simulink model "ramadan_2022"  (R2021a)
settings: Solver=ode15s  StartTime=0.0  StopTime=10  MaxStep=1e-2  MinStep=1e-20  RelTol=1e-3
StartFcn:
  | tic
StopFcn:
  | toc
  | 
  | 
  | %if GimbalLockFlag
  |  % fprintf(2, 'Almost reached Gimbal Lock of IMU. Simulation stopped.\n')
  | %end
  | 
  | %fprintf('Elapsed time: %4.2f sec (%4.2f%% realtime)\n', a, tout(end)/a*100)
values from neighbouring files (symbols this model uses):
  Balance = pMod(26:29)    [AssignSimulinkParams.m]    (also in assign_parameters.m = param(26:29))
  BalanceTrunkLat = pMod(22:25)    [AssignSimulinkParams.m]    (also in assign_parameters.m = param(22:25))
  BasisStim = pMod(1:11)    [AssignSimulinkParams.m]    (also in assign_parameters.m = param(1:11))
  CompliantLeg = pMod(12:14)    [AssignSimulinkParams.m]    (also in assign_parameters.m = param(12:14))
  CompliantLegLat = pMod(15)    [AssignSimulinkParams.m]    (also in assign_parameters.m = param(15))
  lp1 = 0.45    [nms3D_prep.m]
  lp2 = 0.55    [nms3D_prep.m]
  N = size(x,1)    [cmaes_hg.m]
  PreventKneeOverextension = pMod(16:21)    [AssignSimulinkParams.m]    (also in assign_parameters.m = param(16:21))
  propulsion = pMod(35)    [AssignSimulinkParams.m]    (also in assign_parameters.m = param(35))
  s = x(1:N-1,:).^2 + x(2:N,:).^2    [cmaes_hg.m]
  Target02 = pMod(30)    [AssignSimulinkParams.m]    (also in assign_parameters.m = param(30))
  Target13 = pMod(31:33)    [AssignSimulinkParams.m]    (also in assign_parameters.m = param(31:33))
  theta0 = pMod(34)    [AssignSimulinkParams.m]    (also in assign_parameters.m = param(34))
  WramameiSL_1000 = readmatrix('WSL_1000_Norm_Sigmoid_MSE_cont.csv')    [nms3D_prep.m]
  ZramameiSL_1000 = readmatrix('ZSL_1000_Norm_Sigmoid_MSE_cont.csv')    [nms3D_prep.m]
undefined symbols (not defined in the file or in its folder): ICs, mParams, X, Y, Z
libraries: nesl_utility x110, sm_lib x88, simulink x79, eeGeneralControl x28, robotmaniplib x10, dspinverses x10, robotcorelib x5, dspmathops x3, pid_lib x2, vrlib x1
(part 2 of 9)

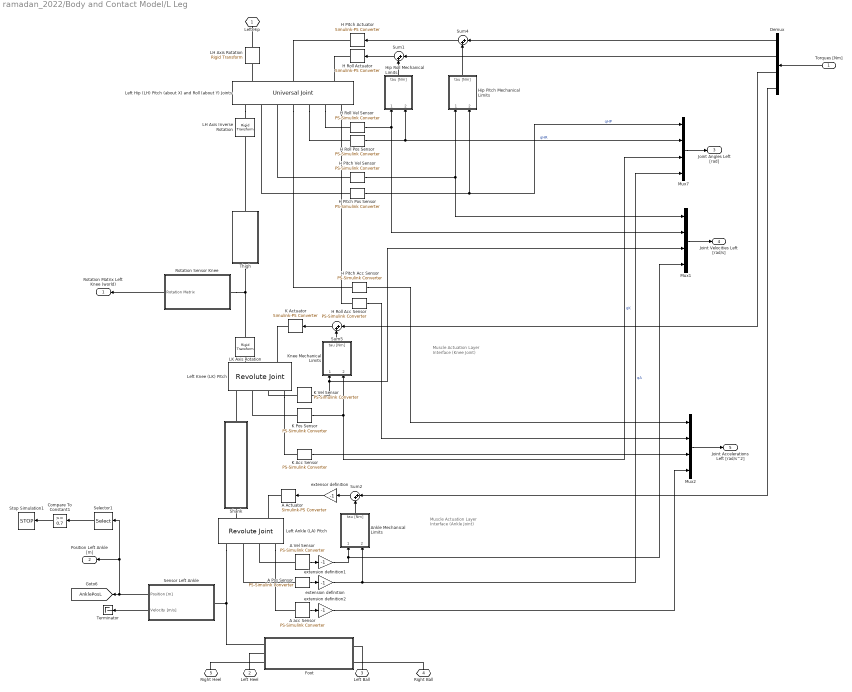
== system ramadan_2022/Body and Contact Model/L Leg ==
  note: Muscle Actuation
      | Layer Interface
      | (Ankle Joint)
  note: Muscle Actuation
      | Layer Interface
      | (Knee Joint)
  Torques [Nm] : Inport
  " K Actuator" : nesl_utility/Simulink-PS Converter  PhysicalDomain=network_engine_domain  SubClassName=ps_input  LeftPortType=input  RightPortType=output  PseudoPeriodic=off  Frequencies=[]  NoiseDistribution=none  NoiseParameters=[]  Unit=N*m  AffineConversion=off  FilteringAndDerivatives=zero  SimscapeFilterOrder=1  InputFilterTimeConstant=.001  UdotUserProvided=0
      settings: SourceProductBaseCode=PW,SS
  A Actuator : nesl_utility/Simulink-PS Converter  PhysicalDomain=network_engine_domain  SubClassName=ps_input  LeftPortType=input  RightPortType=output  PseudoPeriodic=off  Frequencies=[]  NoiseDistribution=none  NoiseParameters=[]  Unit=N*m  AffineConversion=off  FilteringAndDerivatives=zero  SimscapeFilterOrder=1  InputFilterTimeConstant=.001  UdotUserProvided=0
      settings: SourceProductBaseCode=PW,SS
  A Pos Sensor : nesl_utility/PS-Simulink Converter  PhysicalDomain=network_engine_domain  SubClassName=ps_output  LeftPortType=input  RightPortType=output  PseudoPeriodic=off  Frequencies=[]  Unit=rad  AffineConversion=off
      settings: SourceProductBaseCode=PW,SS
  A Vel Sensor : nesl_utility/PS-Simulink Converter  PhysicalDomain=network_engine_domain  SubClassName=ps_output  LeftPortType=input  RightPortType=output  PseudoPeriodic=off  Frequencies=[]  Unit=rad/s  AffineConversion=off
      settings: SourceProductBaseCode=PW,SS
  A acc Sensor : nesl_utility/PS-Simulink Converter  PhysicalDomain=network_engine_domain  SubClassName=ps_output  LeftPortType=input  RightPortType=output  PseudoPeriodic=off  Frequencies=[]  Unit=rad/(s^2)  AffineConversion=off
      settings: SourceProductBaseCode=PW,SS
  Ankle Mechanical Limits : Subsystem
  Compare To Constant1 : simulink/Logic and Bit Operations/Compare To Constant  relop=>=  const=0.7  OutDataTypeStr=boolean
  Demux : Demux
  Foot : Subsystem
  H Pitch Actuator : nesl_utility/Simulink-PS Converter  PhysicalDomain=network_engine_domain  SubClassName=ps_input  LeftPortType=input  RightPortType=output  PseudoPeriodic=off  Frequencies=[]  NoiseDistribution=none  NoiseParameters=[]  Unit=N*m  AffineConversion=off  FilteringAndDerivatives=zero  SimscapeFilterOrder=1  InputFilterTimeConstant=.001  UdotUserProvided=0
      settings: SourceProductBaseCode=PW,SS
  H Pitch Acc Sensor : nesl_utility/PS-Simulink Converter  PhysicalDomain=network_engine_domain  SubClassName=ps_output  LeftPortType=input  RightPortType=output  PseudoPeriodic=off  Frequencies=[]  Unit=rad/(s^2)  AffineConversion=off
      settings: SourceProductBaseCode=PW,SS
  H Pitch Pos Sensor : nesl_utility/PS-Simulink Converter  PhysicalDomain=network_engine_domain  SubClassName=ps_output  LeftPortType=input  RightPortType=output  PseudoPeriodic=off  Frequencies=[]  Unit=rad  AffineConversion=off
      settings: SourceProductBaseCode=PW,SS
  H Pitch Vel Sensor : nesl_utility/PS-Simulink Converter  PhysicalDomain=network_engine_domain  SubClassName=ps_output  LeftPortType=input  RightPortType=output  PseudoPeriodic=off  Frequencies=[]  Unit=rad/s  AffineConversion=off
      settings: SourceProductBaseCode=PW,SS
  H Roll Actuator : nesl_utility/Simulink-PS Converter  PhysicalDomain=network_engine_domain  SubClassName=ps_input  LeftPortType=input  RightPortType=output  PseudoPeriodic=off  Frequencies=[]  NoiseDistribution=none  NoiseParameters=[]  Unit=N*m  AffineConversion=off  FilteringAndDerivatives=zero  SimscapeFilterOrder=1  InputFilterTimeConstant=.001  UdotUserProvided=0
      settings: SourceProductBaseCode=PW,SS
  H Roll Acc Sensor : nesl_utility/PS-Simulink Converter  PhysicalDomain=network_engine_domain  SubClassName=ps_output  LeftPortType=input  RightPortType=output  PseudoPeriodic=off  Frequencies=[]  Unit=rad/(s^2)  AffineConversion=off
      settings: SourceProductBaseCode=PW,SS
  H Roll Pos Sensor : nesl_utility/PS-Simulink Converter  PhysicalDomain=network_engine_domain  SubClassName=ps_output  LeftPortType=input  RightPortType=output  PseudoPeriodic=off  Frequencies=[]  Unit=rad  AffineConversion=off
      settings: SourceProductBaseCode=PW,SS
  "H Roll Vel Sensor " : nesl_utility/PS-Simulink Converter  PhysicalDomain=network_engine_domain  SubClassName=ps_output  LeftPortType=input  RightPortType=output  PseudoPeriodic=off  Frequencies=[]  Unit=rad/s  AffineConversion=off
      settings: SourceProductBaseCode=PW,SS
  Hip Pitch Mechanical Limits : Subsystem
  Hip Roll Mechanical Limits : Subsystem
  K Acc Sensor : nesl_utility/PS-Simulink Converter  PhysicalDomain=network_engine_domain  SubClassName=ps_output  LeftPortType=input  RightPortType=output  PseudoPeriodic=off  Frequencies=[]  Unit=rad/(s^2)  AffineConversion=off
      settings: SourceProductBaseCode=PW,SS
  K Pos Sensor : nesl_utility/PS-Simulink Converter  PhysicalDomain=network_engine_domain  SubClassName=ps_output  LeftPortType=input  RightPortType=output  PseudoPeriodic=off  Frequencies=[]  Unit=rad  AffineConversion=off
      settings: SourceProductBaseCode=PW,SS
  K Vel Sensor : nesl_utility/PS-Simulink Converter  PhysicalDomain=network_engine_domain  SubClassName=ps_output  LeftPortType=input  RightPortType=output  PseudoPeriodic=off  Frequencies=[]  Unit=rad/s  AffineConversion=off
      settings: SourceProductBaseCode=PW,SS
  Knee Mechanical Limits : Subsystem
  LH Axis Inverse Rotation : sm_lib/Frames and Transforms/Rigid Transform  TranslationMethod=None  TranslationStandardOffset=-0.2  TranslationLengthUnit=m  TranslationStandardAxis=+Y  TranslationCartesianOffset=0  TranslationROffset=0  TranslationROffsetUnits=m  TranslationZOffset=0  TranslationZOffsetUnits=m  TranslationThetaOffset=0  TranslationThetaOffsetUnits=deg  RotationMethod=RotationSequence  RotationAngleUnits=deg  RotationStandardAxis=+X  RotationAngle=-90  RotationArbitraryAxis=[0 0 1]  FollAlignAxisA=+X  BaseAlignAxisA=+Y  FollAlignAxisB=+Y  BaseAlignAxisB=+Z  RotationSequenceAxes=BaseAxes  RotationSequence=YXY  RotationSequenceAngles=[-90 -90 0]  RotationSequenceAnglesUnits=deg  RotationMatrix=[1 0 0; 0 1 0; 0 0 1]
  LH Axis Rotation : sm_lib/Frames and Transforms/Rigid Transform  TranslationMethod=None  TranslationStandardOffset=-0.2  TranslationLengthUnit=m  TranslationStandardAxis=+Y  TranslationCartesianOffset=0  TranslationROffset=0  TranslationROffsetUnits=m  TranslationZOffset=0  TranslationZOffsetUnits=m  TranslationThetaOffset=0  TranslationThetaOffsetUnits=deg  RotationMethod=RotationSequence  RotationAngleUnits=deg  RotationStandardAxis=+X  RotationAngle=90  RotationArbitraryAxis=[0 0 1]  FollAlignAxisA=+X  BaseAlignAxisA=+Y  FollAlignAxisB=+Y  BaseAlignAxisB=+Z  RotationSequenceAxes=FollowerAxes  RotationSequence=XZX  RotationSequenceAngles=[-90 90 0]  RotationSequenceAnglesUnits=deg  RotationMatrix=[1 0 0; 0 1 0; 0 0 1]
  LK Axis Rotation : sm_lib/Frames and Transforms/Rigid Transform  TranslationMethod=None  TranslationStandardOffset=-0.5  TranslationLengthUnit=m  TranslationStandardAxis=+Y  TranslationCartesianOffset=0  TranslationROffset=0  TranslationROffsetUnits=m  TranslationZOffset=0  TranslationZOffsetUnits=m  TranslationThetaOffset=0  TranslationThetaOffsetUnits=deg  RotationMethod=RotationSequence  RotationAngleUnits=deg  RotationStandardAxis=+X  RotationAngle=-90  RotationArbitraryAxis=[0 0 1]  FollAlignAxisA=+X  BaseAlignAxisA=+Y  FollAlignAxisB=+Y  BaseAlignAxisB=+Z  RotationSequenceAxes=BaseAxes  RotationSequence=ZXZ  RotationSequenceAngles=[180 0 0]  RotationSequenceAnglesUnits=deg  RotationMatrix=[1 0 0; 0 1 0; 0 0 1]
  Left Ankle (LA) Pitch : sm_lib/Joints/Revolute Joint  JointMode=Normal  SenseConstraintForce=off  SenseConstraintForceX=off  SenseConstraintForceY=off  SenseConstraintForceZ=off  SenseConstraintTorque=off  SenseConstraintTorqueX=off  SenseConstraintTorqueY=off  SenseConstraintTorqueZ=off  SenseTotalForce=off  SenseTotalForceX=off  SenseTotalForceY=off  SenseTotalForceZ=off  SenseTotalTorque=off  SenseTotalTorqueX=off  SenseTotalTorqueY=off  SenseTotalTorqueZ=off  CompositeWrenchDir=FollowerOnBase  CompositeWrenchFrame=FollowerFrame  EquilibriumPosition=0  EquilibriumPositionUnits=deg  SpringStiffness=0  SpringStiffnessUnits=N*m/deg  DampingCoefficient=0  DampingCoefficientUnits=N*m/(deg/s)  TorqueActuationMode=InputTorque  MotionActuationMode=ComputedMotion  SensePosition=on  SenseVelocity=on  SenseAcceleration=on  SenseTorqueForce=off  SenseLowerLimitTorqueForce=off  SenseUpperLimitTorqueForce=off  LowerLimitSpecify=off  LowerLimitBound=-90  LowerLimitBoundUnits=deg  LowerLimitStiffness=1e4  LowerLimitStiffnessUnits=N*m/deg  LowerLimitDamping=10  LowerLimitDampingUnits=N*m/(deg/s)  LowerLimitTransitionRegionWidth=0.1  LowerLimitTransitionRegionWidthUnits=deg  UpperLimitSpecify=off  UpperLimitBound=90  UpperLimitBoundUnits=deg  UpperLimitStiffness=1e4  UpperLimitStiffnessUnits=N*m/deg  UpperLimitDamping=10  UpperLimitDampingUnits=N*m/(deg/s)  UpperLimitTransitionRegionWidth=0.1  UpperLimitTransitionRegionWidthUnits=deg  PositionTargetSpecify=on  PositionTargetPriority=High  PositionTargetValue=-ICs.lLeg.ankle.qP0  PositionTargetValueUnits=rad  VelocityTargetSpecify=on  VelocityTargetPriority=High  VelocityTargetValue=0  VelocityTargetValueUnits=rad/s
  Left Hip (LH) Pitch (about X) and Roll (about Y) Joints : sm_lib/Joints/Universal Joint  JointMode=Normal  SenseConstraintForce=off  SenseConstraintForceX=off  SenseConstraintForceY=off  SenseConstraintForceZ=off  SenseConstraintTorque=off  SenseConstraintTorqueX=off  SenseConstraintTorqueY=off  SenseConstraintTorqueZ=off  SenseTotalForce=off  SenseTotalForceX=off  SenseTotalForceY=off  SenseTotalForceZ=off  SenseTotalTorque=off  SenseTotalTorqueX=off  SenseTotalTorqueY=off  SenseTotalTorqueZ=off  CompositeWrenchDir=FollowerOnBase  CompositeWrenchFrame=FollowerFrame  RxEquilibriumPosition=0  RxEquilibriumPositionUnits=deg  RxSpringStiffness=0  RxSpringStiffnessUnits=N*m/deg  RxDampingCoefficient=0  RxDampingCoefficientUnits=N*m/(deg/s)  RxTorqueActuationMode=InputTorque  RxMotionActuationMode=ComputedMotion  RxSensePosition=on  RxSenseVelocity=on  RxSenseAcceleration=on  RxSenseTorqueForce=off  RxSenseLowerLimitTorqueForce=off  RxSenseUpperLimitTorqueForce=off  RxLowerLimitSpecify=off  RxLowerLimitBound=-90  RxLowerLimitBoundUnits=deg  RxLowerLimitStiffness=1e4  RxLowerLimitStiffnessUnits=N*m/deg  RxLowerLimitDamping=10  RxLowerLimitDampingUnits=N*m/(deg/s)  RxLowerLimitTransitionRegionWidth=0.1  RxLowerLimitTransitionRegionWidthUnits=deg  RxUpperLimitSpecify=off  RxUpperLimitBound=90  RxUpperLimitBoundUnits=deg  RxUpperLimitStiffness=1e4  RxUpperLimitStiffnessUnits=N*m/deg  RxUpperLimitDamping=10  RxUpperLimitDampingUnits=N*m/(deg/s)  RxUpperLimitTransitionRegionWidth=0.1  RxUpperLimitTransitionRegionWidthUnits=deg  RxPositionTargetSpecify=on  RxPositionTargetPriority=High  RxPositionTargetValue=ICs.lLeg.hip.qP0  RxPositionTargetValueUnits=rad  RxVelocityTargetSpecify=on  RxVelocityTargetPriority=High  RxVelocityTargetValue=0  RxVelocityTargetValueUnits=rad/s  RyEquilibriumPosition=0  RyEquilibriumPositionUnits=deg  RySpringStiffness=0  RySpringStiffnessUnits=N*m/deg  RyDampingCoefficient=0  RyDampingCoefficientUnits=N*m/(deg/s)  RyTorqueActuationMode=InputTorque  RyMotionActuationMode=ComputedMotion  RySensePosition=on  RySenseVelocity=on  RySenseAcceleration=on  RySenseTorqueForce=off  RySenseLowerLimitTorqueForce=off  RySenseUpperLimitTorqueForce=off  RyLowerLimitSpecify=off  RyLowerLimitBound=-90  RyLowerLimitBoundUnits=deg  RyLowerLimitStiffness=1e4  RyLowerLimitStiffnessUnits=N*m/deg  RyLowerLimitDamping=10  RyLowerLimitDampingUnits=N*m/(deg/s)  RyLowerLimitTransitionRegionWidth=0.1  RyLowerLimitTransitionRegionWidthUnits=deg  RyUpperLimitSpecify=off  RyUpperLimitBound=90  RyUpperLimitBoundUnits=deg  RyUpperLimitStiffness=1e4  RyUpperLimitStiffnessUnits=N*m/deg  RyUpperLimitDamping=10  RyUpperLimitDampingUnits=N*m/(deg/s)  RyUpperLimitTransitionRegionWidth=0.1  RyUpperLimitTransitionRegionWidthUnits=deg  RyPositionTargetSpecify=on  RyPositionTargetPriority=High  RyPositionTargetValue=ICs.lLeg.hip.qR0  RyPositionTargetValueUnits=rad  RyVelocityTargetSpecify=on  RyVelocityTargetPriority=High  RyVelocityTargetValue=0  RyVelocityTargetValueUnits=rad/s
  Left Knee (LK) Pitch : sm_lib/Joints/Revolute Joint  JointMode=Normal  SenseConstraintForce=off  SenseConstraintForceX=off  SenseConstraintForceY=off  SenseConstraintForceZ=off  SenseConstraintTorque=off  SenseConstraintTorqueX=off  SenseConstraintTorqueY=off  SenseConstraintTorqueZ=off  SenseTotalForce=off  SenseTotalForceX=off  SenseTotalForceY=off  SenseTotalForceZ=off  SenseTotalTorque=off  SenseTotalTorqueX=off  SenseTotalTorqueY=off  SenseTotalTorqueZ=off  CompositeWrenchDir=FollowerOnBase  CompositeWrenchFrame=FollowerFrame  EquilibriumPosition=0  EquilibriumPositionUnits=deg  SpringStiffness=0  SpringStiffnessUnits=N*m/deg  DampingCoefficient=0  DampingCoefficientUnits=N*m/(deg/s)  TorqueActuationMode=InputTorque  MotionActuationMode=ComputedMotion  SensePosition=on  SenseVelocity=on  SenseAcceleration=on  SenseTorqueForce=off  SenseLowerLimitTorqueForce=off  SenseUpperLimitTorqueForce=off  LowerLimitSpecify=off  LowerLimitBound=-90  LowerLimitBoundUnits=deg  LowerLimitStiffness=1e4  LowerLimitStiffnessUnits=N*m/deg  LowerLimitDamping=10  LowerLimitDampingUnits=N*m/(deg/s)  LowerLimitTransitionRegionWidth=0.1  LowerLimitTransitionRegionWidthUnits=deg  UpperLimitSpecify=off  UpperLimitBound=90  UpperLimitBoundUnits=deg  UpperLimitStiffness=1e4  UpperLimitStiffnessUnits=N*m/deg  UpperLimitDamping=10  UpperLimitDampingUnits=N*m/(deg/s)  UpperLimitTransitionRegionWidth=0.1  UpperLimitTransitionRegionWidthUnits=deg  PositionTargetSpecify=on  PositionTargetPriority=High  PositionTargetValue=ICs.lLeg.knee.qP0  PositionTargetValueUnits=rad  VelocityTargetSpecify=on  VelocityTargetPriority=High  VelocityTargetValue=0  VelocityTargetValueUnits=rad/s
  Mux1 : Mux
  Mux2 : Mux
  Mux7 : Mux
  Rotation Sensor Knee : Subsystem
  Selector1 : Selector  InputPortWidth=3  IndexOptions=Index vector (dialog)  Indices=[2]  OutputSizes=1
  Sensor Left Ankle : Subsystem
  Shank : Subsystem
  Stop Simulation1 : Stop
  Sum{1..2,4..5} (4 alike) : Sum  Inputs=|++
  Terminator : Terminator
  Thigh : Subsystem
  extension definition : Gain  Gain=-1
  extension definition1 : Gain  Gain=-1
  extension definition2 : Gain  Gain=-1
  extensor definition : Gain  Gain=-1
  Left Hip : PMIOPort  Side=Left
  Left Heel : PMIOPort  Port=2  Side=Right
  Left Ball : PMIOPort  Port=3  Side=Right
  Right Ball : PMIOPort  Port=4  Side=Right
  Right Heel : PMIOPort  Port=5  Side=Right
  Rotation Matrix Left Knee (world) : Outport
  " Position Left Ankle [m]" : Outport  Port=2
  Joint Angles Left [rad] : Outport  Port=3
  "Joint Velocities Left [rad/s] " : Outport  Port=4
  Joint Accelerations Left [rad/s^2] : Outport  Port=5
  tag scope: AnklePosL=global
  wires:
  extension definition1/1 -> Mux1/4, Ankle Mechanical Limits/1(dq [rad/s])
  A Pos Sensor/1 -> extension definition/1
  Ankle Mechanical Limits/1(tau [Nm]) -> Sum2/2
  A Vel Sensor/1 -> extension definition1/1
  Sum2/1 -> extensor definition/1
  "H Roll Vel Sensor "/1 -> Mux1/2, Hip Roll Mechanical Limits/1(dq [rad/s])
  K Vel Sensor/1 -> Mux1/3, Knee Mechanical Limits/1(dq [rad/s])
  Knee Mechanical Limits/1(tau [Nm]) -> Sum5/2
  Hip Roll Mechanical Limits/1(tau [Nm]) -> Sum1/2
  H Pitch Vel Sensor/1 -> Mux1/1, Hip Pitch Mechanical Limits/1(dq [rad/s])
  Hip Pitch Mechanical Limits/1(tau [Nm]) -> Sum4/2
  Sum4/1 -> H Pitch Actuator/1
  Sum1/1 -> H Roll Actuator/1
  Sum5/1 -> " K Actuator"/1
  extensor definition/1 -> A Actuator/1
  Mux1/1 -> "Joint Velocities Left [rad/s] "/1
  Mux2/1 -> Joint Accelerations Left [rad/s^2]/1
  H Pitch Acc Sensor/1 -> Mux2/1
  H Roll Acc Sensor/1 -> Mux2/2
  K Acc Sensor/1 -> Mux2/3
  A acc Sensor/1 -> extension definition2/1
  extension definition2/1 -> Mux2/4
  Demux/1 -> Sum4/1
  Demux/2 -> Sum1/1
  Demux/3 -> Sum5/1
  Demux/4 -> Sum2/1
  Sensor Left Ankle/1(Position [m]) -> " Position Left Ankle [m]"/1, Selector1/1, [AnklePosL]
  Rotation Sensor Knee/1(Rotation Matrix) -> Rotation Matrix Left Knee (world)/1
  Sensor Left Ankle/2(Velocity [m/s]) -> Terminator/1
  Torques [Nm]/1 -> Demux/1
  K Pos Sensor/1 -> Mux7/3, Knee Mechanical Limits/2(q [rad])  "qK"
  H Pitch Pos Sensor/1 -> Hip Pitch Mechanical Limits/2(q [rad]), Mux7/1  "qHP"
  H Roll Pos Sensor/1 -> Mux7/2, Hip Roll Mechanical Limits/2(q [rad])  "qHR"
  extension definition/1 -> Mux7/4, Ankle Mechanical Limits/2(q [rad])  "qA"
  Mux7/1 -> Joint Angles Left [rad]/1
  Selector1/1 -> Compare To Constant1/1
  Compare To Constant1/1 -> Stop Simulation1/1
  connections:
  Left Ankle (LA) Pitch/RConn1 -- Sensor Left Ankle/LConn1 -- Foot/LConn1
  A Pos Sensor/LConn1 -- Left Ankle (LA) Pitch/RConn2
  A Vel Sensor/LConn1 -- Left Ankle (LA) Pitch/RConn3
  Left Ankle (LA) Pitch/LConn1 -- Shank/RConn1
  Left Hip (LH) Pitch (about X) and Roll (about Y) Joints/RConn1 -- LH Axis Inverse Rotation/LConn1
  Thigh/RConn1 -- Rotation Sensor Knee/LConn1 -- LK Axis Rotation/LConn1
  Shank/LConn1 -- Left Knee (LK) Pitch/RConn1
  Left Hip (LH) Pitch (about X) and Roll (about Y) Joints/LConn1 -- LH Axis Rotation/RConn1
  H Pitch Vel Sensor/LConn1 -- Left Hip (LH) Pitch (about X) and Roll (about Y) Joints/RConn3
  H Pitch Pos Sensor/LConn1 -- Left Hip (LH) Pitch (about X) and Roll (about Y) Joints/RConn2
  K Pos Sensor/LConn1 -- Left Knee (LK) Pitch/RConn2
  K Vel Sensor/LConn1 -- Left Knee (LK) Pitch/RConn3
  LH Axis Rotation/LConn1 -- Left Hip/RConn1
  Left Hip (LH) Pitch (about X) and Roll (about Y) Joints/RConn6 -- "H Roll Vel Sensor "/LConn1
  Left Hip (LH) Pitch (about X) and Roll (about Y) Joints/RConn5 -- H Roll Pos Sensor/LConn1
  Left Hip (LH) Pitch (about X) and Roll (about Y) Joints/RConn4 -- H Pitch Acc Sensor/LConn1
  Left Hip (LH) Pitch (about X) and Roll (about Y) Joints/RConn7 -- H Roll Acc Sensor/LConn1
  Left Knee (LK) Pitch/RConn4 -- K Acc Sensor/LConn1
  Left Ankle (LA) Pitch/RConn4 -- A acc Sensor/LConn1
  LK Axis Rotation/RConn1 -- Left Knee (LK) Pitch/LConn1
  Right Heel/RConn1 -- Foot/LConn3
  Foot/LConn2 -- Left Heel/RConn1
  Left Ball/RConn1 -- Foot/RConn1
  Right Ball/RConn1 -- Foot/RConn2
  Thigh/LConn1 -- LH Axis Inverse Rotation/RConn1
  " K Actuator"/RConn1 -- Left Knee (LK) Pitch/LConn2
  A Actuator/RConn1 -- Left Ankle (LA) Pitch/LConn2
  H Pitch Actuator/RConn1 -- Left Hip (LH) Pitch (about X) and Roll (about Y) Joints/LConn2
  H Roll Actuator/RConn1 -- Left Hip (LH) Pitch (about X) and Roll (about Y) Joints/LConn3

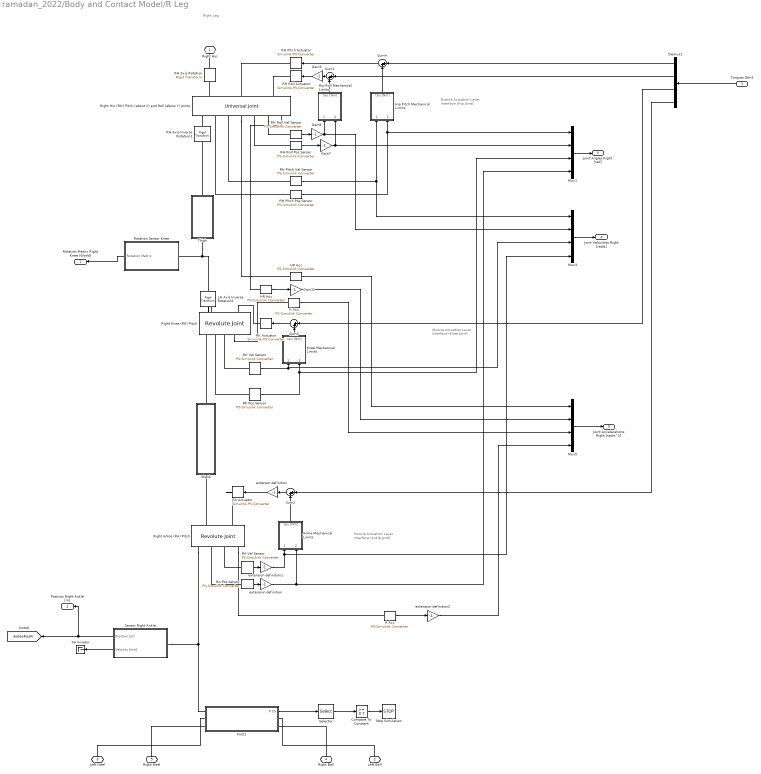
== system ramadan_2022/Body and Contact Model/R Leg ==
  note: Muscle Actuation
      | Layer Interface
      | (Hip Joint)
  note: Muscle Actuation
      | Layer Interface
      | (Knee Joint)
  note: Muscle Actuation
      | Layer Interface
      | (Ankle Joint)
  note: Right Leg
  Torques [Nm] : Inport
  A Acc : nesl_utility/PS-Simulink Converter  PhysicalDomain=network_engine_domain  SubClassName=ps_output  LeftPortType=input  RightPortType=output  PseudoPeriodic=off  Frequencies=[]  Unit=rad/(s^2)  AffineConversion=off
      settings: SourceProductBaseCode=PW,SS
  Ankle Mechanical Limits : Subsystem
  Compare To Constant : simulink/Logic and Bit Operations/Compare To Constant  relop=>=  const=0.7  OutDataTypeStr=boolean
  Demux1 : Demux
  Foot1 : Subsystem
  Gain{3,7..8,11} (4 alike) : Gain  Gain=-1
  HP Acc : nesl_utility/PS-Simulink Converter  PhysicalDomain=network_engine_domain  SubClassName=ps_output  LeftPortType=input  RightPortType=output  PseudoPeriodic=off  Frequencies=[]  Unit=rad/(s^2)  AffineConversion=off
      settings: SourceProductBaseCode=PW,SS
  HR Acc : nesl_utility/PS-Simulink Converter  PhysicalDomain=network_engine_domain  SubClassName=ps_output  LeftPortType=input  RightPortType=output  PseudoPeriodic=off  Frequencies=[]  Unit=rad/(s^2)  AffineConversion=off
      settings: SourceProductBaseCode=PW,SS
  Hip Pitch Mechanical Limits : Subsystem
  Hip Roll Mechanical Limits : Subsystem
  K Acc : nesl_utility/PS-Simulink Converter  PhysicalDomain=network_engine_domain  SubClassName=ps_output  LeftPortType=input  RightPortType=output  PseudoPeriodic=off  Frequencies=[]  Unit=rad/(s^2)  AffineConversion=off
      settings: SourceProductBaseCode=PW,SS
  Knee Mechanical Limits : Subsystem
  LH Axis Inverse Rotation1 : sm_lib/Frames and Transforms/Rigid Transform  TranslationMethod=None  TranslationStandardOffset=-0.5  TranslationLengthUnit=m  TranslationStandardAxis=+Y  TranslationCartesianOffset=0  TranslationROffset=0  TranslationROffsetUnits=m  TranslationZOffset=0  TranslationZOffsetUnits=m  TranslationThetaOffset=0  TranslationThetaOffsetUnits=deg  RotationMethod=RotationSequence  RotationAngleUnits=deg  RotationStandardAxis=+X  RotationAngle=-90  RotationArbitraryAxis=[0 0 1]  FollAlignAxisA=+X  BaseAlignAxisA=+Y  FollAlignAxisB=+Y  BaseAlignAxisB=+Z  RotationSequenceAxes=BaseAxes  RotationSequence=ZXZ  RotationSequenceAngles=[180 0 0]  RotationSequenceAnglesUnits=deg  RotationMatrix=[1 0 0; 0 1 0; 0 0 1]
  Mux1 : Mux
  Mux3 : Mux
  Mux5 : Mux
  RA Actuator : nesl_utility/Simulink-PS Converter  PhysicalDomain=network_engine_domain  SubClassName=ps_input  LeftPortType=input  RightPortType=output  PseudoPeriodic=off  Frequencies=[]  NoiseDistribution=none  NoiseParameters=[]  Unit=N*m  AffineConversion=off  FilteringAndDerivatives=zero  SimscapeFilterOrder=1  InputFilterTimeConstant=.001  UdotUserProvided=0
      settings: SourceProductBaseCode=PW,SS
  RA Pos Sensor : nesl_utility/PS-Simulink Converter  PhysicalDomain=network_engine_domain  SubClassName=ps_output  LeftPortType=input  RightPortType=output  PseudoPeriodic=off  Frequencies=[]  Unit=rad  AffineConversion=off
      settings: SourceProductBaseCode=PW,SS
  RA Vel Sensor : nesl_utility/PS-Simulink Converter  PhysicalDomain=network_engine_domain  SubClassName=ps_output  LeftPortType=input  RightPortType=output  PseudoPeriodic=off  Frequencies=[]  Unit=rad/s  AffineConversion=off
      settings: SourceProductBaseCode=PW,SS
  RH Pitch Pos Sensor : nesl_utility/PS-Simulink Converter  PhysicalDomain=network_engine_domain  SubClassName=ps_output  LeftPortType=input  RightPortType=output  PseudoPeriodic=off  Frequencies=[]  Unit=rad  AffineConversion=off
      settings: SourceProductBaseCode=PW,SS
  RH Pitch Vel Sensor : nesl_utility/PS-Simulink Converter  PhysicalDomain=network_engine_domain  SubClassName=ps_output  LeftPortType=input  RightPortType=output  PseudoPeriodic=off  Frequencies=[]  Unit=rad/s  AffineConversion=off
      settings: SourceProductBaseCode=PW,SS
  RH Roll Pos Sensor : nesl_utility/PS-Simulink Converter  PhysicalDomain=network_engine_domain  SubClassName=ps_output  LeftPortType=input  RightPortType=output  PseudoPeriodic=off  Frequencies=[]  Unit=rad  AffineConversion=off
      settings: SourceProductBaseCode=PW,SS
  "RH Roll Vel Sensor " : nesl_utility/PS-Simulink Converter  PhysicalDomain=network_engine_domain  SubClassName=ps_output  LeftPortType=input  RightPortType=output  PseudoPeriodic=off  Frequencies=[]  Unit=rad/s  AffineConversion=off
      settings: SourceProductBaseCode=PW,SS
  RH Axis Inverse Rotation1 : sm_lib/Frames and Transforms/Rigid Transform  TranslationMethod=None  TranslationStandardOffset=-0.5  TranslationLengthUnit=m  TranslationStandardAxis=+Y  TranslationCartesianOffset=[0 0.2 0]  TranslationROffset=0  TranslationROffsetUnits=m  TranslationZOffset=0  TranslationZOffsetUnits=m  TranslationThetaOffset=0  TranslationThetaOffsetUnits=deg  RotationMethod=RotationSequence  RotationAngleUnits=deg  RotationStandardAxis=+X  RotationAngle=-90  RotationArbitraryAxis=[0 0 1]  FollAlignAxisA=+X  BaseAlignAxisA=+Y  FollAlignAxisB=+Y  BaseAlignAxisB=+Z  RotationSequenceAxes=BaseAxes  RotationSequence=YXY  RotationSequenceAngles=[ -90 -90 0]  RotationSequenceAnglesUnits=deg  RotationMatrix=[1 0 0; 0 1 0; 0 0 1]
  RH Axis Rotation : sm_lib/Frames and Transforms/Rigid Transform  TranslationMethod=None  TranslationStandardOffset=-0  TranslationLengthUnit=m  TranslationStandardAxis=+Y  TranslationCartesianOffset=0  TranslationROffset=0  TranslationROffsetUnits=m  TranslationZOffset=0  TranslationZOffsetUnits=m  TranslationThetaOffset=0  TranslationThetaOffsetUnits=deg  RotationMethod=RotationSequence  RotationAngleUnits=deg  RotationStandardAxis=+X  RotationAngle=90  RotationArbitraryAxis=[0 0 1]  FollAlignAxisA=+X  BaseAlignAxisA=+Y  FollAlignAxisB=+Y  BaseAlignAxisB=+Z  RotationSequenceAxes=FollowerAxes  RotationSequence=XZX  RotationSequenceAngles=[-90 90 0]  RotationSequenceAnglesUnits=deg  RotationMatrix=[1 0 0; 0 1 0; 0 0 1]
  RH Pitch Actuator : nesl_utility/Simulink-PS Converter  PhysicalDomain=network_engine_domain  SubClassName=ps_input  LeftPortType=input  RightPortType=output  PseudoPeriodic=off  Frequencies=[]  NoiseDistribution=none  NoiseParameters=[]  Unit=N*m  AffineConversion=off  FilteringAndDerivatives=zero  SimscapeFilterOrder=1  InputFilterTimeConstant=.001  UdotUserProvided=0
      settings: SourceProductBaseCode=PW,SS
  RH Roll Actuator : nesl_utility/Simulink-PS Converter  PhysicalDomain=network_engine_domain  SubClassName=ps_input  LeftPortType=input  RightPortType=output  PseudoPeriodic=off  Frequencies=[]  NoiseDistribution=none  NoiseParameters=[]  Unit=N*m  AffineConversion=off  FilteringAndDerivatives=zero  SimscapeFilterOrder=1  InputFilterTimeConstant=.001  UdotUserProvided=0
      settings: SourceProductBaseCode=PW,SS
  RK Actuator : nesl_utility/Simulink-PS Converter  PhysicalDomain=network_engine_domain  SubClassName=ps_input  LeftPortType=input  RightPortType=output  PseudoPeriodic=off  Frequencies=[]  NoiseDistribution=none  NoiseParameters=[]  Unit=N*m  AffineConversion=off  FilteringAndDerivatives=zero  SimscapeFilterOrder=1  InputFilterTimeConstant=.001  UdotUserProvided=0
      settings: SourceProductBaseCode=PW,SS
  RK Pos Sensor : nesl_utility/PS-Simulink Converter  PhysicalDomain=network_engine_domain  SubClassName=ps_output  LeftPortType=input  RightPortType=output  PseudoPeriodic=off  Frequencies=[]  Unit=rad  AffineConversion=off
      settings: SourceProductBaseCode=PW,SS
  RK Vel Sensor : nesl_utility/PS-Simulink Converter  PhysicalDomain=network_engine_domain  SubClassName=ps_output  LeftPortType=input  RightPortType=output  PseudoPeriodic=off  Frequencies=[]  Unit=rad/s  AffineConversion=off
      settings: SourceProductBaseCode=PW,SS
  Right Ankle (RA) Pitch : sm_lib/Joints/Revolute Joint  JointMode=Normal  SenseConstraintForce=off  SenseConstraintForceX=off  SenseConstraintForceY=off  SenseConstraintForceZ=off  SenseConstraintTorque=off  SenseConstraintTorqueX=off  SenseConstraintTorqueY=off  SenseConstraintTorqueZ=off  SenseTotalForce=off  SenseTotalForceX=off  SenseTotalForceY=off  SenseTotalForceZ=off  SenseTotalTorque=off  SenseTotalTorqueX=off  SenseTotalTorqueY=off  SenseTotalTorqueZ=off  CompositeWrenchDir=FollowerOnBase  CompositeWrenchFrame=FollowerFrame  EquilibriumPosition=0  EquilibriumPositionUnits=deg  SpringStiffness=0  SpringStiffnessUnits=N*m/deg  DampingCoefficient=0  DampingCoefficientUnits=N*m/(deg/s)  TorqueActuationMode=InputTorque  MotionActuationMode=ComputedMotion  SensePosition=on  SenseVelocity=on  SenseAcceleration=on  SenseTorqueForce=off  SenseLowerLimitTorqueForce=off  SenseUpperLimitTorqueForce=off  LowerLimitSpecify=off  LowerLimitBound=-90  LowerLimitBoundUnits=deg  LowerLimitStiffness=1e4  LowerLimitStiffnessUnits=N*m/deg  LowerLimitDamping=10  LowerLimitDampingUnits=N*m/(deg/s)  LowerLimitTransitionRegionWidth=0.1  LowerLimitTransitionRegionWidthUnits=deg  UpperLimitSpecify=off  UpperLimitBound=90  UpperLimitBoundUnits=deg  UpperLimitStiffness=1e4  UpperLimitStiffnessUnits=N*m/deg  UpperLimitDamping=10  UpperLimitDampingUnits=N*m/(deg/s)  UpperLimitTransitionRegionWidth=0.1  UpperLimitTransitionRegionWidthUnits=deg  PositionTargetSpecify=on  PositionTargetPriority=High  PositionTargetValue=-ICs.rLeg.ankle.qP0  PositionTargetValueUnits=rad  VelocityTargetSpecify=on  VelocityTargetPriority=High  VelocityTargetValue=0  VelocityTargetValueUnits=rad/s
  Right Hip (RH) Pitch (about X) and Roll (about Y) Joints : sm_lib/Joints/Universal Joint  JointMode=Normal  SenseConstraintForce=off  SenseConstraintForceX=off  SenseConstraintForceY=off  SenseConstraintForceZ=off  SenseConstraintTorque=off  SenseConstraintTorqueX=off  SenseConstraintTorqueY=off  SenseConstraintTorqueZ=off  SenseTotalForce=off  SenseTotalForceX=off  SenseTotalForceY=off  SenseTotalForceZ=off  SenseTotalTorque=off  SenseTotalTorqueX=off  SenseTotalTorqueY=off  SenseTotalTorqueZ=off  CompositeWrenchDir=FollowerOnBase  CompositeWrenchFrame=FollowerFrame  RxEquilibriumPosition=0  RxEquilibriumPositionUnits=deg  RxSpringStiffness=0  RxSpringStiffnessUnits=N*m/deg  RxDampingCoefficient=0  RxDampingCoefficientUnits=N*m/(deg/s)  RxTorqueActuationMode=InputTorque  RxMotionActuationMode=ComputedMotion  RxSensePosition=on  RxSenseVelocity=on  RxSenseAcceleration=on  RxSenseTorqueForce=off  RxSenseLowerLimitTorqueForce=off  RxSenseUpperLimitTorqueForce=off  RxLowerLimitSpecify=off  RxLowerLimitBound=-90  RxLowerLimitBoundUnits=deg  RxLowerLimitStiffness=1e4  RxLowerLimitStiffnessUnits=N*m/deg  RxLowerLimitDamping=10  RxLowerLimitDampingUnits=N*m/(deg/s)  RxLowerLimitTransitionRegionWidth=0.1  RxLowerLimitTransitionRegionWidthUnits=deg  RxUpperLimitSpecify=off  RxUpperLimitBound=90  RxUpperLimitBoundUnits=deg  RxUpperLimitStiffness=1e4  RxUpperLimitStiffnessUnits=N*m/deg  RxUpperLimitDamping=10  RxUpperLimitDampingUnits=N*m/(deg/s)  RxUpperLimitTransitionRegionWidth=0.1  RxUpperLimitTransitionRegionWidthUnits=deg  RxPositionTargetSpecify=on  RxPositionTargetPriority=High  RxPositionTargetValue=ICs.rLeg.hip.qP0  RxPositionTargetValueUnits=rad  RxVelocityTargetSpecify=on  RxVelocityTargetPriority=High  RxVelocityTargetValue=0  RxVelocityTargetValueUnits=rad/s  RyEquilibriumPosition=0  RyEquilibriumPositionUnits=deg  RySpringStiffness=0  RySpringStiffnessUnits=N*m/deg  RyDampingCoefficient=0  RyDampingCoefficientUnits=N*m/(deg/s)  RyTorqueActuationMode=InputTorque  RyMotionActuationMode=ComputedMotion  RySensePosition=on  RySenseVelocity=on  RySenseAcceleration=on  RySenseTorqueForce=off  RySenseLowerLimitTorqueForce=off  RySenseUpperLimitTorqueForce=off  RyLowerLimitSpecify=off  RyLowerLimitBound=-90  RyLowerLimitBoundUnits=deg  RyLowerLimitStiffness=1e4  RyLowerLimitStiffnessUnits=N*m/deg  RyLowerLimitDamping=10  RyLowerLimitDampingUnits=N*m/(deg/s)  RyLowerLimitTransitionRegionWidth=0.1  RyLowerLimitTransitionRegionWidthUnits=deg  RyUpperLimitSpecify=off  RyUpperLimitBound=90  RyUpperLimitBoundUnits=deg  RyUpperLimitStiffness=1e4  RyUpperLimitStiffnessUnits=N*m/deg  RyUpperLimitDamping=10  RyUpperLimitDampingUnits=N*m/(deg/s)  RyUpperLimitTransitionRegionWidth=0.1  RyUpperLimitTransitionRegionWidthUnits=deg  RyPositionTargetSpecify=on  RyPositionTargetPriority=High  RyPositionTargetValue=-ICs.rLeg.hip.qR0  RyPositionTargetValueUnits=rad  RyVelocityTargetSpecify=on  RyVelocityTargetPriority=High  RyVelocityTargetValue=0  RyVelocityTargetValueUnits=rad/s
  Right Knee (RK) Pitch : sm_lib/Joints/Revolute Joint  JointMode=Normal  SenseConstraintForce=off  SenseConstraintForceX=off  SenseConstraintForceY=off  SenseConstraintForceZ=off  SenseConstraintTorque=off  SenseConstraintTorqueX=off  SenseConstraintTorqueY=off  SenseConstraintTorqueZ=off  SenseTotalForce=off  SenseTotalForceX=off  SenseTotalForceY=off  SenseTotalForceZ=off  SenseTotalTorque=off  SenseTotalTorqueX=off  SenseTotalTorqueY=off  SenseTotalTorqueZ=off  CompositeWrenchDir=FollowerOnBase  CompositeWrenchFrame=FollowerFrame  EquilibriumPosition=0  EquilibriumPositionUnits=deg  SpringStiffness=0  SpringStiffnessUnits=N*m/deg  DampingCoefficient=0  DampingCoefficientUnits=N*m/(deg/s)  TorqueActuationMode=InputTorque  MotionActuationMode=ComputedMotion  SensePosition=on  SenseVelocity=on  SenseAcceleration=on  SenseTorqueForce=on  SenseLowerLimitTorqueForce=off  SenseUpperLimitTorqueForce=off  LowerLimitSpecify=off  LowerLimitBound=-90  LowerLimitBoundUnits=deg  LowerLimitStiffness=1e4  LowerLimitStiffnessUnits=N*m/deg  LowerLimitDamping=10  LowerLimitDampingUnits=N*m/(deg/s)  LowerLimitTransitionRegionWidth=0.1  LowerLimitTransitionRegionWidthUnits=deg  UpperLimitSpecify=off  UpperLimitBound=90  UpperLimitBoundUnits=deg  UpperLimitStiffness=1e4  UpperLimitStiffnessUnits=N*m/deg  UpperLimitDamping=10  UpperLimitDampingUnits=N*m/(deg/s)  UpperLimitTransitionRegionWidth=0.1  UpperLimitTransitionRegionWidthUnits=deg  PositionTargetSpecify=on  PositionTargetPriority=High  PositionTargetValue=ICs.rLeg.knee.qP0  PositionTargetValueUnits=rad  VelocityTargetSpecify=on  VelocityTargetPriority=High  VelocityTargetValue=0  VelocityTargetValueUnits=rad/s
  Rotation Sensor Knee : Subsystem
  Selector : Selector  InputPortWidth=3  IndexOptions=Index vector (dialog)  Indices=[2]  OutputSizes=1
  Sensor Right Ankle : Subsystem
  Shank : Subsystem
  Stop Simulation : Stop
  Sum{1..2,4..5} (4 alike) : Sum  Inputs=|++
  Terminator : Terminator
  Thigh : Subsystem
  extension definition : Gain  Gain=-1
  extension definition1 : Gain  Gain=-1
  extension definition2 : Gain  Gain=-1
  extensor definition : Gain  Gain=-1
  Right Hip : PMIOPort  Side=Left
  "Left Ball " : PMIOPort  Port=2  Side=Right
  Left Heel : PMIOPort  Port=3  Side=Right
  Right Ball : PMIOPort  Port=4  Side=Right
  Right Heel : PMIOPort  Port=5  Side=Right
  Rotation Matrix Right Knee (World) : Outport
  Position Right Ankle [m] : Outport  Port=2
  Joint Angles Right [rad] : Outport  Port=3
  "Joint Velocities Right [rad/s] " : Outport  Port=4
  Joint Accelerations Right [rad/s^2] : Outport  Port=5
  tag scope: AnklePosR=global
  wires:
  Hip Pitch Mechanical Limits/1(tau [Nm]) -> Sum4/2
  RH Pitch Vel Sensor/1 -> Mux3/1, Hip Pitch Mechanical Limits/1(dq [rad/s])
  Hip Roll Mechanical Limits/1(tau [Nm]) -> Sum1/2
  RK Pos Sensor/1 -> Knee Mechanical Limits/2(q [rad]), Mux1/3
  Demux1/3 -> Sum5/1
  RK Vel Sensor/1 -> Mux3/3, Knee Mechanical Limits/1(dq [rad/s])
  RH Pitch Pos Sensor/1 -> Hip Pitch Mechanical Limits/2(q [rad]), Mux1/1
  RH Roll Pos Sensor/1 -> Gain7/1
  Demux1/1 -> Sum4/1
  Sum2/1 -> extensor definition/1
  RA Vel Sensor/1 -> extension definition1/1
  Demux1/4 -> Sum2/1
  Ankle Mechanical Limits/1(tau [Nm]) -> Sum2/2
  RA Pos Sensor/1 -> extension definition/1
  extension definition/1 -> Mux1/4, Ankle Mechanical Limits/2(q [rad])
  extension definition1/1 -> Mux3/4, Ankle Mechanical Limits/1(dq [rad/s])
  Sum4/1 -> RH Pitch Actuator/1
  Sum1/1 -> Gain3/1
  Gain3/1 -> RH Roll Actuator/1
  Sum5/1 -> RK Actuator/1
  extensor definition/1 -> RA Actuator/1
  "RH Roll Vel Sensor "/1 -> Gain8/1
  Gain8/1 -> Mux3/2, Hip Roll Mechanical Limits/1(dq [rad/s])
  Gain7/1 -> Mux1/2, Hip Roll Mechanical Limits/2(q [rad])
  Demux1/2 -> Sum1/1
  Mux3/1 -> "Joint Velocities Right [rad/s] "/1
  Mux5/1 -> Joint Accelerations Right [rad/s^2]/1
  HP Acc/1 -> Mux5/1
  HR Acc/1 -> Gain11/1
  Gain11/1 -> Mux5/2
  K Acc/1 -> Mux5/3
  A Acc/1 -> extension definition2/1
  extension definition2/1 -> Mux5/4
  Knee Mechanical Limits/1(tau [Nm]) -> Sum5/2
  Sensor Right Ankle/1(Position [m]) -> Position Right Ankle [m]/1, [AnklePosR]
  Rotation Sensor Knee/1(Rotation Matrix) -> Rotation Matrix Right Knee (World)/1
  Selector/1 -> Compare To Constant/1
  Compare To Constant/1 -> Stop Simulation/1
  Foot1/1(P CG) -> Selector/1
  Sensor Right Ankle/2(Velocity [m/s]) -> Terminator/1
  Torques [Nm]/1 -> Demux1/1
  Mux1/1 -> Joint Angles Right [rad]/1
  connections:
  RH Axis Rotation/LConn1 -- Right Hip/RConn1
  RK Vel Sensor/LConn1 -- Right Knee (RK) Pitch/RConn3
  RK Pos Sensor/LConn1 -- Right Knee (RK) Pitch/RConn2
  RH Pitch Pos Sensor/LConn1 -- Right Hip (RH) Pitch (about X) and Roll (about Y) Joints/RConn2
  RH Pitch Vel Sensor/LConn1 -- Right Hip (RH) Pitch (about X) and Roll (about Y) Joints/RConn3
  Right Hip (RH) Pitch (about X) and Roll (about Y) Joints/LConn1 -- RH Axis Rotation/RConn1
  Shank/LConn1 -- Right Knee (RK) Pitch/RConn1
  LH Axis Inverse Rotation1/RConn1 -- Right Knee (RK) Pitch/LConn1
  Right Ankle (RA) Pitch/LConn1 -- Shank/RConn1
  RA Vel Sensor/LConn1 -- Right Ankle (RA) Pitch/RConn3
  RA Pos Sensor/LConn1 -- Right Ankle (RA) Pitch/RConn2
  RH Axis Inverse Rotation1/LConn1 -- Right Hip (RH) Pitch (about X) and Roll (about Y) Joints/RConn1
  Right Hip (RH) Pitch (about X) and Roll (about Y) Joints/RConn5 -- RH Roll Pos Sensor/LConn1
  Right Hip (RH) Pitch (about X) and Roll (about Y) Joints/RConn6 -- "RH Roll Vel Sensor "/LConn1
  Right Hip (RH) Pitch (about X) and Roll (about Y) Joints/RConn4 -- HP Acc/LConn1
  Right Hip (RH) Pitch (about X) and Roll (about Y) Joints/RConn7 -- HR Acc/LConn1
  Right Knee (RK) Pitch/RConn4 -- K Acc/LConn1
  Right Ankle (RA) Pitch/RConn4 -- A Acc/LConn1
  Right Heel/RConn1 -- Foot1/LConn3
  Left Heel/RConn1 -- Foot1/LConn2
  Right Ball/RConn1 -- Foot1/RConn2
  "Left Ball "/RConn1 -- Foot1/RConn1
  Thigh/LConn1 -- RH Axis Inverse Rotation1/RConn1
  Thigh/RConn1 -- LH Axis Inverse Rotation1/LConn1 -- Rotation Sensor Knee/LConn1
  Right Ankle (RA) Pitch/RConn1 -- Sensor Right Ankle/LConn1 -- Foot1/LConn1
  RK Actuator/RConn1 -- Right Knee (RK) Pitch/LConn2
  RA Actuator/RConn1 -- Right Ankle (RA) Pitch/LConn2
  RH Pitch Actuator/RConn1 -- Right Hip (RH) Pitch (about X) and Roll (about Y) Joints/LConn2
  RH Roll Actuator/RConn1 -- Right Hip (RH) Pitch (about X) and Roll (about Y) Joints/LConn3

== system ramadan_2022/Body and Contact Model/Sensor Left Ankle ==
  note: Position and Velocity Sensor in World Frame
  Frame Sensor : sm_lib/Frames and Transforms/Transform Sensor  MeasurementFrame=Base  SenseAngle=off  SenseAxis=off  SenseAngle1=off  SenseAngle2=off  SenseAngle3=off  SenseQ=off  SenseR=off  SenseOmegaX=off  SenseOmegaY=off  SenseOmegaZ=off  SenseOmega1=off  SenseOmega2=off  SenseOmega3=off  SenseQDot=off  SenseRDot=off  SenseAlphaX=off  SenseAlphaY=off  SenseAlphaZ=off  SenseAlpha1=off  SenseAlpha2=off  SenseAlpha3=off  SenseQDDot=off  SenseRDDot=off  SenseX=on  SenseY=on  SenseZ=on  SenseRad=off  SenseAzim=off  SenseDist=off  SenseInc=off  SenseXDot=on  SenseYDot=on  SenseZDot=on  SenseRadDot=off  SenseAzimDot=off  SenseDistDot=off  SenseIncDot=off  SenseXDDot=off  SenseYDDot=off  SenseZDDot=off  SenseRadDDot=off  SenseAzimDDot=off  SenseDistDDot=off  SenseIncDDot=off
  Mux : Mux  Inputs=3
  Mux1 : Mux  Inputs=3
  PS-Simulink Converter1 : nesl_utility/PS-Simulink Converter  PhysicalDomain=network_engine_domain  SubClassName=ps_output  LeftPortType=input  RightPortType=output  PseudoPeriodic=off  Frequencies=[]  Unit=m  AffineConversion=off
      settings: SourceProductBaseCode=PW,SS
  PS-Simulink Converter12 : nesl_utility/PS-Simulink Converter  PhysicalDomain=network_engine_domain  SubClassName=ps_output  LeftPortType=input  RightPortType=output  PseudoPeriodic=off  Frequencies=[]  Unit=m  AffineConversion=off
      settings: SourceProductBaseCode=PW,SS
  PS-Simulink Converter2 : nesl_utility/PS-Simulink Converter  PhysicalDomain=network_engine_domain  SubClassName=ps_output  LeftPortType=input  RightPortType=output  PseudoPeriodic=off  Frequencies=[]  Unit=m  AffineConversion=off
      settings: SourceProductBaseCode=PW,SS
  PS-Simulink Converter3 : nesl_utility/PS-Simulink Converter  PhysicalDomain=network_engine_domain  SubClassName=ps_output  LeftPortType=input  RightPortType=output  PseudoPeriodic=off  Frequencies=[]  Unit=m/s  AffineConversion=off
      settings: SourceProductBaseCode=PW,SS
  PS-Simulink Converter4 : nesl_utility/PS-Simulink Converter  PhysicalDomain=network_engine_domain  SubClassName=ps_output  LeftPortType=input  RightPortType=output  PseudoPeriodic=off  Frequencies=[]  Unit=m/s  AffineConversion=off
      settings: SourceProductBaseCode=PW,SS
  PS-Simulink Converter5 : nesl_utility/PS-Simulink Converter  PhysicalDomain=network_engine_domain  SubClassName=ps_output  LeftPortType=input  RightPortType=output  PseudoPeriodic=off  Frequencies=[]  Unit=m/s  AffineConversion=off
      settings: SourceProductBaseCode=PW,SS
  World Frame : sm_lib/Frames and Transforms/World Frame
  Frame : PMIOPort  Side=Left
  Position [m] : Outport  VectorParamsAs1DForOutWhenUnconnected=off
  Velocity [m/s] : Outport  Port=2  VectorParamsAs1DForOutWhenUnconnected=off
  wires:
  PS-Simulink Converter12/1 -> Mux/1
  PS-Simulink Converter1/1 -> Mux/2
  PS-Simulink Converter2/1 -> Mux/3
  Mux/1 -> Position [m]/1
  PS-Simulink Converter5/1 -> Mux1/3
  PS-Simulink Converter4/1 -> Mux1/1
  Mux1/1 -> Velocity [m/s]/1
  PS-Simulink Converter3/1 -> Mux1/2
  connections:
  Frame Sensor/RConn1 -- Frame/RConn1
  PS-Simulink Converter12/LConn1 -- Frame Sensor/RConn2
  Frame Sensor/RConn3 -- PS-Simulink Converter1/LConn1
  Frame Sensor/RConn4 -- PS-Simulink Converter2/LConn1
  Frame Sensor/RConn7 -- PS-Simulink Converter5/LConn1
  Frame Sensor/RConn5 -- PS-Simulink Converter4/LConn1
  Frame Sensor/RConn6 -- PS-Simulink Converter3/LConn1
  World Frame/RConn1 -- Frame Sensor/LConn1

== system ramadan_2022/Body and Contact Model/Sensor Left Ankle1 ==
  note: Position and Velocity Sensor in World Frame
  Frame Sensor : sm_lib/Frames and Transforms/Transform Sensor  MeasurementFrame=Base  SenseAngle=off  SenseAxis=off  SenseAngle1=off  SenseAngle2=off  SenseAngle3=off  SenseQ=off  SenseR=off  SenseOmegaX=off  SenseOmegaY=off  SenseOmegaZ=off  SenseOmega1=off  SenseOmega2=off  SenseOmega3=off  SenseQDot=off  SenseRDot=off  SenseAlphaX=off  SenseAlphaY=off  SenseAlphaZ=off  SenseAlpha1=off  SenseAlpha2=off  SenseAlpha3=off  SenseQDDot=off  SenseRDDot=off  SenseX=on  SenseY=on  SenseZ=on  SenseRad=off  SenseAzim=off  SenseDist=off  SenseInc=off  SenseXDot=on  SenseYDot=on  SenseZDot=on  SenseRadDot=off  SenseAzimDot=off  SenseDistDot=off  SenseIncDot=off  SenseXDDot=off  SenseYDDot=off  SenseZDDot=off  SenseRadDDot=off  SenseAzimDDot=off  SenseDistDDot=off  SenseIncDDot=off
  Mux : Mux  Inputs=3
  Mux1 : Mux  Inputs=3
  PS-Simulink Converter1 : nesl_utility/PS-Simulink Converter  PhysicalDomain=network_engine_domain  SubClassName=ps_output  LeftPortType=input  RightPortType=output  PseudoPeriodic=off  Frequencies=[]  Unit=m  AffineConversion=off
      settings: SourceProductBaseCode=PW,SS
  PS-Simulink Converter12 : nesl_utility/PS-Simulink Converter  PhysicalDomain=network_engine_domain  SubClassName=ps_output  LeftPortType=input  RightPortType=output  PseudoPeriodic=off  Frequencies=[]  Unit=m  AffineConversion=off
      settings: SourceProductBaseCode=PW,SS
  PS-Simulink Converter2 : nesl_utility/PS-Simulink Converter  PhysicalDomain=network_engine_domain  SubClassName=ps_output  LeftPortType=input  RightPortType=output  PseudoPeriodic=off  Frequencies=[]  Unit=m  AffineConversion=off
      settings: SourceProductBaseCode=PW,SS
  PS-Simulink Converter3 : nesl_utility/PS-Simulink Converter  PhysicalDomain=network_engine_domain  SubClassName=ps_output  LeftPortType=input  RightPortType=output  PseudoPeriodic=off  Frequencies=[]  Unit=m/s  AffineConversion=off
      settings: SourceProductBaseCode=PW,SS
  PS-Simulink Converter4 : nesl_utility/PS-Simulink Converter  PhysicalDomain=network_engine_domain  SubClassName=ps_output  LeftPortType=input  RightPortType=output  PseudoPeriodic=off  Frequencies=[]  Unit=m/s  AffineConversion=off
      settings: SourceProductBaseCode=PW,SS
  PS-Simulink Converter5 : nesl_utility/PS-Simulink Converter  PhysicalDomain=network_engine_domain  SubClassName=ps_output  LeftPortType=input  RightPortType=output  PseudoPeriodic=off  Frequencies=[]  Unit=m/s  AffineConversion=off
      settings: SourceProductBaseCode=PW,SS
  World Frame : sm_lib/Frames and Transforms/World Frame
  Frame : PMIOPort  Side=Left
  Position [m] : Outport  VectorParamsAs1DForOutWhenUnconnected=off
  Velocity [m/s] : Outport  Port=2  VectorParamsAs1DForOutWhenUnconnected=off
  wires:
  PS-Simulink Converter12/1 -> Mux/1
  PS-Simulink Converter1/1 -> Mux/2
  PS-Simulink Converter2/1 -> Mux/3
  Mux/1 -> Position [m]/1
  PS-Simulink Converter5/1 -> Mux1/3
  PS-Simulink Converter4/1 -> Mux1/1
  Mux1/1 -> Velocity [m/s]/1
  PS-Simulink Converter3/1 -> Mux1/2
  connections:
  Frame Sensor/RConn1 -- Frame/RConn1
  PS-Simulink Converter12/LConn1 -- Frame Sensor/RConn2
  Frame Sensor/RConn3 -- PS-Simulink Converter1/LConn1
  Frame Sensor/RConn4 -- PS-Simulink Converter2/LConn1
  Frame Sensor/RConn7 -- PS-Simulink Converter5/LConn1
  Frame Sensor/RConn5 -- PS-Simulink Converter4/LConn1
  Frame Sensor/RConn6 -- PS-Simulink Converter3/LConn1
  World Frame/RConn1 -- Frame Sensor/LConn1
